simulink model "Correlation_Ex3"  (R2024a)
settings: Solver=VariableStepAuto  StartTime=0.0  StopTime=2048/100e6  RelTol=1e-3
undefined symbols (not defined in the file): S, vsva2197, xcvc1902
libraries: aieDSP x1, vmcUtilities x1
settings Model: Creator=sdegala  LastModifiedBy=robg
settings ModelReferenceCC: EnableRefExpFcnMdlSchedulingChecks=on
settings RTWCC: GPUComputeCapability=3.5

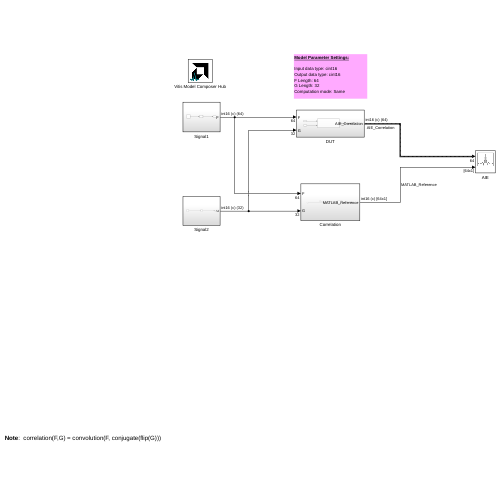
[thumbnail: Simulink's stored preview of the top-level diagram]
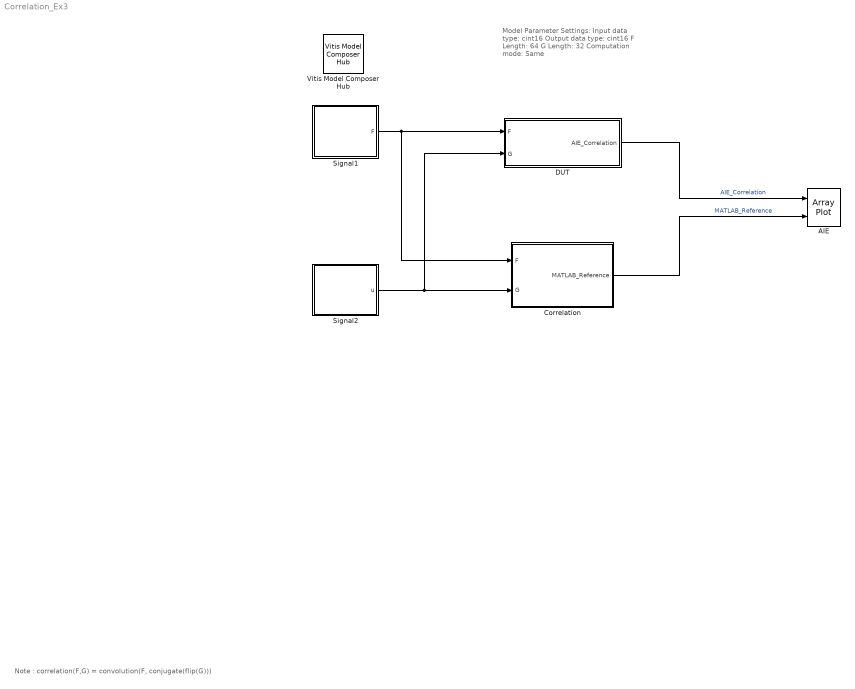
== system Correlation_Ex3 ==
  note: Note : correlation(F,G) = convolution(F, conjugate(flip(G))​)
  note: Model Parameter Settings:
      |
      | Input data type: cint16
      | Output data type: cint16
      | F Length: 64
      | G Length: 32
      | Computation mode: Same
  AIE : ArrayPlot  NumInputPorts=2  WindowPosition=[864.000000,100.000000,800.000000,500.000000,]  ScopeFrameLocation=window  YLimits=[-135.125 86.125]  ShowLegend=on
  Correlation : Subsystem
  DUT : Subsystem
  Signal1 : Subsystem
  Signal2 : Subsystem
  Vitis Model Composer Hub : vmcUtilities/Vitis Model Composer Hub  Tag=genX  CodeGeneration=off  StartColumn=1  NumberOfColumns=1  TargetDirectory=./code  exportDesign=off  analyzeDesign=off  validateDesignOnHw=off  ExportType=AI Engines  IpVendor=xilinx.com  IpLibrary=hls  IpVersion=1.0  IpHWLanguage=Verilog  AieCompilerOptions={}  AieSimulatorOptions={}  CreateTestbench=off  TestbenchStackSize=10  RunRtlSim=off  RunCSim=off  RunAieSim=off  AieSimTimeout=50000  RunAieSimProfiling=off  LaunchVitisAnalyzer=off  PlotOutput=off  RunX86Sim=off  X86SimTimeout=10  GenHwImage=off  GenLibadfXo=off  GenHwValidationCode=off  PlatformType=Not Specified  HwSystemType=Baremetal  HwValidationTarget=hw  ProjDevice=xcvc1902-vsva2197-1LP-e-S  ProjDevicePart=xcvc1902-vsva2197-1LP-e-S  AIEType=AIE  SamplePeriod=-1  ClockFrequency=200  DataPathParallelism=1  xilinxfamily=versalaicore  part=xcvc1902  speed=-1LP-e-S  package=vsva2197  directory=./netlist  testbench=off  incr_netlist=off  synthesis_tool=Vivado  clock_wrapper=Clock Enables  dbl_ovrd=According to Block Masks  dcm_input_clock_period=10  sysclk_period=10  simulink_period=1  eval_field=0  LogFileName=''  NThreads=4
  wires:
  Signal2/1(u) -> DUT/2(G), Correlation/2(G)
  DUT/1(AIE_Correlation) -> AIE/1  "AIE_Correlation"
  Signal1/1(F) -> DUT/1(F), Correlation/1(F)
  Correlation/1(MATLAB_Reference) -> AIE/2  "MATLAB_Reference"

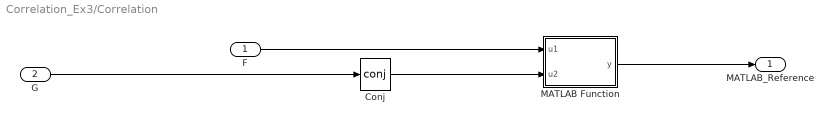
== system Correlation_Ex3/Correlation ==
  F : Inport
  G : Inport  Port=2
  Conj : Math  Operator=conj
  MATLAB Function : MATLAB Function  TreatAsAtomicUnit=on
  MATLAB_Reference : Outport
  wires:
  G/1 -> Conj/1
  F/1 -> MATLAB Function/1(u1)
  MATLAB Function/1(y) -> MATLAB_Reference/1
  Conj/1 -> MATLAB Function/2(u2)

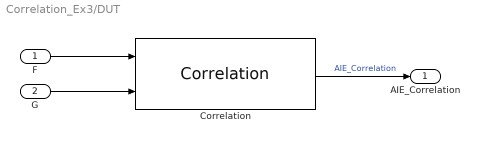
== system Correlation_Ex3/DUT ==
  F : Inport
  G : Inport  Port=2
  Correlation : aieDSP/Correlation  AIE_VARIANT=1  api=0  data_type_f=cint16  data_type_g=cint16  data_type_out=cint16  function_type=0  compute_mode=Same  f_sample_size=64  g_sample_size=32  USE_RTP_VECTOR_LENGTHS=off  num_frames=1  shift_output=0  rnd_mode=Floor  sat_mode=None  no_of_kernels=1  casc_length=1  blockJsonConstraints=[]  blockJsonConstraintsInternal=[]  spec=vmc_corr.json  SerializedMaskParamNames=[]  SerializedMaskParamValues=[]  SerializedMaskParamVisibilities=[]  block_type=Correlation  SerializedMaskParamDataypes=uint|uint|typename|typename|typename|uint|uint|uint|uint|uint|uint|uint|uint|uint|uint|uint  SerializedMaskParamEnumStrArr=0|0|0|0|0|0|Full,Same,Valid|0|0|0|0|0|Floor,Ceiling,Round to positive infinity,Round to negative infinity,Round symmetrical to infinity,Round symmetrical to zero,Round convergent to even,Round convergent to odd|None,Saturate,Symmetric|0|0  SerializedMaskParamEnumValArr=0|0|0|0|0|0|0,1,2|0|0|0|0|0|0,1,2,3,4,5,6,7|0,1,3|0|0  SerializedMaskParamVectorArr=0|0|0|0|0|0|0|0|0|0|0|0|0|0|0|0  SerializedMaskParamKeys=AIE_VARIANT|TP_API|TT_DATA_F|TT_DATA_G|TT_DATA_OUT|TP_FUNCT_TYPE|TP_COMPUTE_MODE|TP_F_LEN|TP_G_LEN|TP_USE_RTP_VECTOR_LENGTHS|TP_NUM_FRAMES|TP_SHIFT|TP_RND|TP_SAT|TP_PHASES|TP_CASC_LEN
  AIE_Correlation : Outport
  wires:
  F/1 -> Correlation/1
  G/1 -> Correlation/2
  Correlation/1 -> AIE_Correlation/1  "AIE_Correlation"

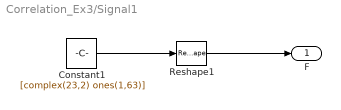
== system Correlation_Ex3/Signal1 ==
  Constant1 : Constant  Value=[complex(23,2) ones(1,63)]  OutDataTypeStr=int16  SampleTime=1/100e6
  Reshape1 : Reshape
  F : Outport
  wires:
  Reshape1/1 -> F/1
  Constant1/1 -> Reshape1/1

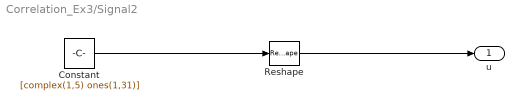
== system Correlation_Ex3/Signal2 ==
  Constant : Constant  Value=[complex(1,5) ones(1,31)]  OutDataTypeStr=int16  SampleTime=1/100e6
  Reshape : Reshape
  u : Outport
  wires:
  Reshape/1 -> u/1
  Constant/1 -> Reshape/1

== matlab function Correlation_Ex3/Correlation/MATLAB Function ==
  data: u1 input; y output; u2 input
function y = func(u1,u2)

y = int16(conv(u1,flip(u2),'same'));
